simulink model "Experiment_cs"  (R2019a)
settings: Solver=ode5  StartTime=0.0  StopTime=inf  FixedStep=1/20  RelTol=1e-3
PreLoadFcn:
  | mbxruntime.callbacks.PreLoadFcn(bdroot);
PostLoadFcn:
  | mbxruntime.callbacks.PostLoadFcn(bdroot);
InitFcn:
  | mbxruntime.callbacks.InitFcn(bdroot);
StartFcn:
  | mbxruntime.callbacks.StartFcn(bdroot);
StopFcn:
  | mbxruntime.callbacks.StopFcn(bdroot);
model workspace: external: MAT-File .\Experiment_cs_hws.mat (data not in the file)
undefined symbols (not defined in the file or in its folder): DiscIntNeverNeededParam, Experiment_cs_BMW_X5_SUV_1_Dynamics_Empty_STATE_BMW_X5_SUV_1_x0, Experiment_cs_BMW_X5_SUV_1_Dynamics_Empty_STATE_BMW_X5_SUV_1_y0, Experiment_cs_BMW_X5_SUV_1_Dynamics_Empty_STATE_BMW_X5_SUV_1_z0, Experiment_cs_e1d584482631291c, Experiment_cs_e726c63043403dc7, Experiment_cs_f4cae83923a86e0b, InitImageOutputDir
libraries: adeye_lib x26, PreScanSimulinkLibrary x2, robotlib x1, PreScanUsefulBlocks x1
(part 1 of 2)
CloseFcn:
  | mbxruntime.callbacks.CloseFcn(bdroot);
settings Model: Creator=PRESCAN  LastModifiedBy=adeye
settings DataIOCC: LimitDataPoints=on  SaveFormat=Array  SignalLoggingSaveFormat=ModelDataLogs  ReturnWorkspaceOutputs=off
settings OptimizationCC: DefaultParameterBehavior=Inlined  ExpressionDepthLimit=2147483647  InitFltsAndDblsToZero=on  LifeSpan=inf
settings DebuggingCC: SaveWithParameterizedLinksMsg=none  UnderspecifiedInitializationDetection=Classic  MergeDetectMultiDrivingBlocksExec=none  SignalResolutionControl=TryResolveAllWithWarning  MultiTaskDSMMsg=warning  MultiTaskCondExecSysMsg=none  FcnCallInpInsideContextMsg=warning  StateNameClashWarn=warning  SFUnexpectedBacktrackingDiag=warning  SFNoUnconditionalDefaultTransitionDiag=warning  SFExecutionAtInitializationDiag=none  ArithmeticOperatorsInVariantConditions=warning
settings HardwareCC: ProdBitPerPointer=32  ProdBitPerSizeT=32  ProdBitPerPtrDiffT=32  ProdLargestAtomicFloat=None  ProdIntDivRoundTo=Undefined  ProdEndianess=Unspecified  ProdWordSize=32  ProdHWDeviceType=32-bit Generic
settings ModelReferenceCC: UpdateModelReferenceTargets=IfOutOfDate  PropagateSignalLabelsOutOfModel=off
settings SFSimCC: SimUseLocalCustomCode=off  SimParseCustomCode=off
settings SFSimCC: SimCustomHeaderCode=|
  | #include "prescan.h"
  | #include "prescan_platform.h"
settings RTWCC: RTWUseLocalCustomCode=off
settings CodeAppCC: StateflowObjectComments=on
settings GRTTargetCC: TargetFcnLib=ansi_tfl_tmw.mat  TargetLangStandard=C89/C90 (ANSI)  GeneratePreprocessorConditionals=Disable all  CombineOutputUpdateFcns=off  GRTInterface=on
settings ConfigComp: CovMetricSettings=dw  CovHtmlReporting=on  CovSaveCumulativeToWorkspaceVar=on  CovSaveSingleToWorkspaceVar=on  CovExternalEMLEnable=off  CovSFcnEnable=off

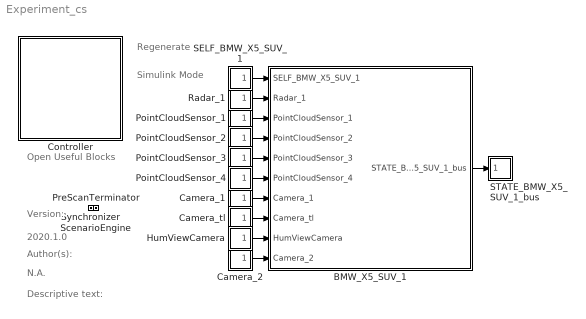
== system Experiment_cs ==
  note: Regenerate
  note: Simulink Mode
  note: Open Useful Blocks
  note: 2020.1.0
  note: Version:
  note: Author(s):
  note: N.A.
  note: Descriptive text:
  BMW_X5_SUV_1 : Subsystem  Tag=WorldObjectSubSystem  InitFcn=UniqueId = '256';
      mask init:
      | modelPath = GenericModelHelper.getGenericModelFilePath('ModelDepo','Vehicles\BMW_X5\BMW_X5.pgmb','bfeb1c11467705ab888b3011684c848b');imagePath = GenericModelHelper.getCompilationPicture(modelPath, 'BMW_X5_HighPoly.png');
      mask Display: image(imread(imagePath));color('white');text(0, 0, ' ID=14\n')
  Camera_1 : Subsystem  Tag=sensor/Camera/CameraSensor  Priority=30  mask(PreScan Source Block: Camera Sensor){}
      mask help: The Camera Sensor provides a color or monochrome image.
      settings: OpenFcn=open_system([gcb '/Sensor'],'mask')
      mask Help: eval('openHelp(457)')
      mask Display: image(imread('CameraSensor.png'))
  Camera_2 : Subsystem  Tag=sensor/Camera/CameraSensor  Priority=30  mask(PreScan Source Block: Camera Sensor){}
      mask help: The Camera Sensor provides a color or monochrome image.
      settings: OpenFcn=open_system([gcb '/Sensor'],'mask')
      mask Help: eval('openHelp(457)')
      mask Display: image(imread('CameraSensor.png'))
  Camera_tl : Subsystem  Tag=sensor/Camera/CameraSensor  Priority=30  mask(PreScan Source Block: Camera Sensor){}
      mask help: The Camera Sensor provides a color or monochrome image.
      settings: OpenFcn=open_system([gcb '/Sensor'],'mask')
      mask Help: eval('openHelp(457)')
      mask Display: image(imread('CameraSensor.png'))
  Controller : Subsystem  Description=8A3CD2955739A82C886C20AE3E253D78460D53180EE2C1B14CC08DF75A70BE77  Priority=-1  LoadFcn=load PreScanControllerData  mask(PreScan Simulation Controller){prescanversion='2020.1.0', ModelReferencing=off, TimeStep=1/20, ControlMode=0, PreScanExecutionMode=on, ControllerCount=0, ControllerIndex=0, ControllerOptions=''}
      mask prompts: prescanversion "PreScan Version"; ModelReferencing "Use Model Referencing"; TimeStep "Upload Period [s]"; ControlMode "Control Mode"; PreScanExecutionMode "Execution Mode"; ControllerCount "Controller Count"; ControllerIndex "Controller Index"; ControllerOptions "Controller Options"
      mask help:
      | Please do not remove this block from the compilation sheet,
      | as it connects the model to the PreScan environment.
      mask init:
      | model = bdroot(gcb);
      | ExperimentFile = mbxruntime.findExperimentFile(model,true); %relative path
      | 
      | [d1, d2, d3, prescandata] = prescan_Settings();
      | ModelDepo = fullfile(prescandata,'ModelDepo'); 
      | 
      | RTmode = mbxruntime.getRTMode(model);
      | 
      | SimulationMode = get_param(bdroot,'SimulationMode');
      | if strcmp(SimulationMode, 'rapid-accelerator')
      |     SimulationMode = 'external';
      | end
      | TargetName = get_param(bdroot,'SystemTargetFile');
      settings: ModelCloseFcn=assignin('base',['model_closed_' bdroot],true);
      mask Help: eval('openHelp(812)')
      mask Display: image(imread('prescanlogo.ico'))
  HumViewCamera : Subsystem  Tag=sensor/Camera/CameraSensor  Priority=30  mask(PreScan Source Block: Camera Sensor){}
      mask help: The Camera Sensor provides a color or monochrome image.
      settings: OpenFcn=open_system([gcb '/Sensor'],'mask')
      mask Help: eval('openHelp(457)')
      mask Display: image(imread('CameraSensor.png'))
  PointCloudSensor_1 : Subsystem  Tag=sensor/PointCloudInport  Priority=30  mask(PreScan Source Block: Point Cloud Sensor){}
      mask help: The Point Cloud Sensor provides XYZ positions relative to the sensor
      settings: OpenFcn=open_system([gcb '/Sensor'],'mask')
      mask Help: eval('openHelp(6400)')
      mask Display: image(imread('PointCloudSensorSL.png'))
  PointCloudSensor_2 : Subsystem  Tag=sensor/PointCloudInport  Priority=30  mask(PreScan Source Block: Point Cloud Sensor){}
      mask help: The Point Cloud Sensor provides XYZ positions relative to the sensor
      settings: OpenFcn=open_system([gcb '/Sensor'],'mask')
      mask Help: eval('openHelp(6400)')
      mask Display: image(imread('PointCloudSensorSL.png'))
  PointCloudSensor_3 : Subsystem  Tag=sensor/PointCloudInport  Priority=30  mask(PreScan Source Block: Point Cloud Sensor){}
      mask help: The Point Cloud Sensor provides XYZ positions relative to the sensor
      settings: OpenFcn=open_system([gcb '/Sensor'],'mask')
      mask Help: eval('openHelp(6400)')
      mask Display: image(imread('PointCloudSensorSL.png'))
  PointCloudSensor_4 : Subsystem  Tag=sensor/PointCloudInport  Priority=30  mask(PreScan Source Block: Point Cloud Sensor){}
      mask help: The Point Cloud Sensor provides XYZ positions relative to the sensor
      settings: OpenFcn=open_system([gcb '/Sensor'],'mask')
      mask Help: eval('openHelp(6400)')
      mask Display: image(imread('PointCloudSensorSL.png'))
  PreScanTerminator : Subsystem  Tag=PreScanTerminator  Priority=999  LoadFcn=load PrescanTerminatorData  mask(PreScan Simulation Terminator){TimeStep=1/20}
      mask prompts: TimeStep "Upload Period [s]"
      mask help:
      | Please do not remove this block from the compilation sheet as it
      | connects the model to the PreScan environment.
      mask Help: eval('openHelp(812)')
      mask Display: image(imread('prescanlogo.ico'))
  Radar_1 : Subsystem  Tag=sensor/Radar  Priority=30  LoadFcn=load('PrescanScannerSensorData.mat');load('PrescanScannerSensorMessage.mat')  mask(PreScan Source Block: Radar Sensor){}
      mask help:
      | The Radar Sensor is a detailed sensor based on a physical radar
      | model that includes Antenna GAIN Maps (AGM) and atmospheric
      | attenuation.
      |
      | For more information, please click Help.
      settings: OpenFcn=open_system([gcb '/Sensor'],'mask')
      mask Help: eval('openHelp(1464)')
      mask Display: image(imread('Radar.png'))
  SELF_BMW_X5_SUV_1 : Subsystem  Tag=sensor/SelfPort  Priority=30  LoadFcn=load('PreScanSelfSensorData.mat')  mask(PreScan Source Block: SELF){}
      mask help:
      | The SELF port shows (state) information of the actor itself. The outputs are position in the experiment's axis system and the GPS coordinates, and the object's absolute velocity and compass heading.
      |
      | For more information, please click Help.
      settings: OpenFcn=open_system([gcb '/Sensor'],'mask')
      mask Help: eval('openHelp(462)')
      mask Display: image(imread('GPS.png'))
  STATE_BMW_X5_SUV_1_bus : Subsystem  Tag=actuator/StatePort  Priority=0  LoadFcn=load('PreScanStateActuatorData.mat')  mask(PreScan Sink Block: State){}
      mask help:
      | The Actor State contains a vector signal of size (9x1), containing the following signals:
      |
      | -  Position    	(x,y,z)             	[m]
      | -  Velocity    	(vx,vy,vz)         	[m/s]
      | -  Angles       	(Roll, Pitch, Yaw)	[rad]
      |
      | The Actor state is defined in the global axis system.
      | The state is superponed on the Initial position defined in the GUI.
      |
      | For more information, please click Help.
      settings: OpenFcn=open_system([gcb '/Actuator'],'mask')
      mask Help: eval('openHelp(222)')
      mask Display: image(imread('State.png'))
  ScenarioEngine : Subsystem  Tag=PreScanOpenScenarioBlock  Priority=10  LoadFcn=load PrescanSynchronizeData  mask(PreScan Simulation Core Block){TimeStep=1/20}
      mask prompts: TimeStep "Timestep [s]"
      mask help:
      | Please do not remove this block from the PreScan compilation sheet,
      | as it contains essential configuration parameters for a PreScan simulation.
      settings: DeleteFcn=PreScanBlockDeleteFcn;
      mask Display: image(imread('prescanlogo.ico'))
  Synchronizer : Subsystem  Tag=PreScanSynchronizer  Priority=20  LoadFcn=load PrescanSynchronizeData  mask(PreScan Simulation Core Block){TimeStep=1/20}
      mask prompts: TimeStep "Timestep [s]"
      mask help:
      | Please do not remove this block from the PreScan compilation sheet,
      | as it contains essential configuration parameters for a PreScan simulation.
      settings: DeleteFcn=PreScanBlockDeleteFcn;
      mask Display: image(imread('prescanlogo.ico'))
  wires:
  BMW_X5_SUV_1/1(STATE_BMW_X5_SUV_1_bus) -> STATE_BMW_X5_SUV_1_bus/1(STATE_BMW_X5_SUV_1_bus)
  SELF_BMW_X5_SUV_1/1(SELF_BMW_X5_SUV_1) -> BMW_X5_SUV_1/1(SELF_BMW_X5_SUV_1)
  Radar_1/1(Radar_1) -> BMW_X5_SUV_1/2(Radar_1)
  PointCloudSensor_1/1(PointCloudSensor_1) -> BMW_X5_SUV_1/3(PointCloudSensor_1)
  PointCloudSensor_2/1(PointCloudSensor_2) -> BMW_X5_SUV_1/4(PointCloudSensor_2)
  PointCloudSensor_3/1(PointCloudSensor_3) -> BMW_X5_SUV_1/5(PointCloudSensor_3)
  PointCloudSensor_4/1(PointCloudSensor_4) -> BMW_X5_SUV_1/6(PointCloudSensor_4)
  Camera_1/1(Camera_1) -> BMW_X5_SUV_1/7(Camera_1)
  Camera_tl/1(Camera_tl) -> BMW_X5_SUV_1/8(Camera_tl)
  HumViewCamera/1(HumViewCamera) -> BMW_X5_SUV_1/9(HumViewCamera)
  Camera_2/1(Camera_2) -> BMW_X5_SUV_1/10(Camera_2)

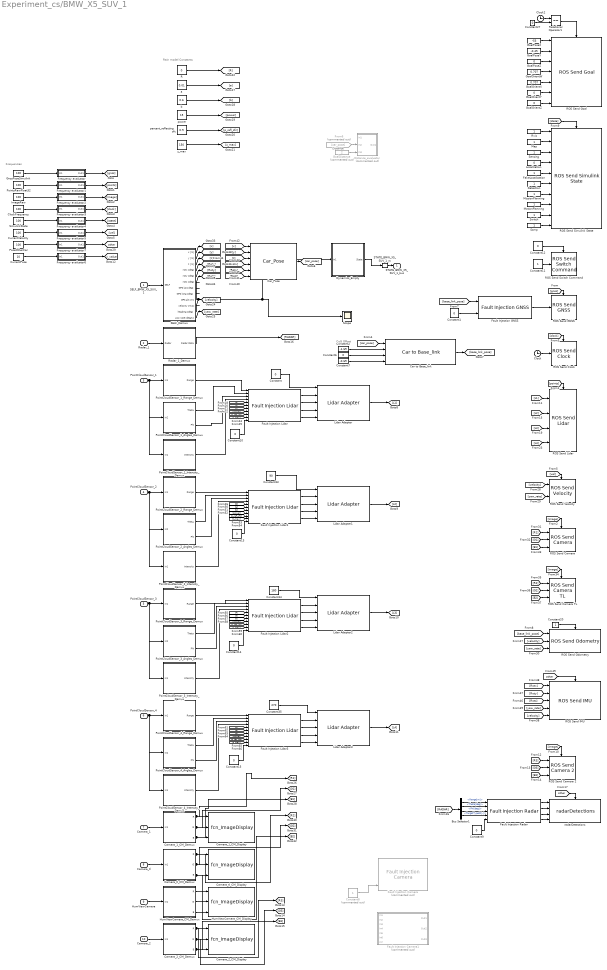
== system Experiment_cs/BMW_X5_SUV_1 ==
  note: Distance
  note: Frequencies
  note: CoG Offset
  note: Rain model Constants
  SELF_BMW_X5_SUV_1 : Inport  Tag=inport/SelfPort  OutDataTypeStr=Bus: PRESCAN_SELFSENSORDATA  PortDimensions=1  SampleTime=1/20  BusOutputAsStruct=on
  Radar_1 : Inport  Tag=inport/Radar  Port=2  OutDataTypeStr=Bus: PRESCAN_SCANNERSENSOR_MESSAGE  PortDimensions=7  SampleTime=1/20  BusOutputAsStruct=on
  PointCloudSensor_1 : Inport  Tag=inport/PointCloudInport  Port=3  OutDataTypeStr=single  SampleTime=1/20  BusOutputAsStruct=on
  PointCloudSensor_2 : Inport  Tag=inport/PointCloudInport  Port=4  OutDataTypeStr=single  SampleTime=1/20  BusOutputAsStruct=on
  PointCloudSensor_3 : Inport  Tag=inport/PointCloudInport  Port=5  OutDataTypeStr=single  SampleTime=1/20  BusOutputAsStruct=on
  PointCloudSensor_4 : Inport  Tag=inport/PointCloudInport  Port=6  OutDataTypeStr=single  SampleTime=1/20  BusOutputAsStruct=on
  Camera_1 : Inport  Tag=inport/Camera/CameraSensor  Port=7  OutDataTypeStr=uint8  SampleTime=1/20  BusOutputAsStruct=on
  Camera_tl : Inport  Tag=inport/Camera/CameraSensor  Port=8  OutDataTypeStr=uint8  SampleTime=1/20  BusOutputAsStruct=on
  HumViewCamera : Inport  Tag=inport/Camera/CameraSensor  Port=9  OutDataTypeStr=uint8  SampleTime=1/20  BusOutputAsStruct=on
  Camera_2 : Inport  Tag=inport/Camera/CameraSensor  Port=10  OutDataTypeStr=uint8  SampleTime=1/20  BusOutputAsStruct=on
  Bus Selector1 : BusSelector  OutputSignals=Range[m],Theta[deg],Phi[deg],TargetTypeID[-]
  Camera_1_CM_Demux : Subsystem  Tag=demux/Camera/Color  mask{SensorName=Camera_1, hres=960, vres=720}
      mask prompts: SensorName "Sensor Name"; hres "Horizontal Resolution"; vres "Vertical Resolution"
      mask Help: eval('openHelp(457)')
      mask Display:
      | fprintf('MONO CAMERA:\n Color\n %s \n %d x %d px',SensorName,hres,vres)
      | port_label('output',1,'R')
      | port_label('output',2,'G')
      | port_label('output',3,'B')
  Camera_1_CM_Display : M-S-Function  Tag=CameraSensor_Color_Display  InitFcn=InitImageOutputDir(gcb);  FunctionName=fcn_ImageDisplay  Parameters=SensorName EnableDisplay EnablePosition DisplayPosition FigureHandle SaveResults BitmapFormat TempOutputDir CameraType DataType  mask(PreScan Color Display Block){SensorName=Camera_1, EnableDisplay=on, EnablePosition=off, DisplayPosition=[10 10 960 720], FigureHandle=25605, SaveResults=off, Format=PNG, TempOutputDir=0, CameraType=Mono, DataType=uint8}
      mask prompts: SensorName "User Specified: Title of Display"; EnableDisplay "Active"; EnablePosition "Set Display window position"; DisplayPosition "Display window position [xpos ypos width height]"; FigureHandle "Unique Handle"; SaveResults "Save results"; TempOutputDir "OutputDir"; CameraType "Camera Type"; DataType "Image Data Type"
      mask help: This block displays the RGB output of a PreScan camera sensor.
      mask init:
      | if EnableDisplay
      |     EnableString='';
      |     EnableColor='gray';
      | else
      |     EnableString='INACTIVE';
      |     EnableColor='red';
      | end
      | switch Format
      |     case 1
      |         BitmapFormat = 'png';
      |     case 2
      |         BitmapFormat = 'bmp';
      |     case 3
      |         BitmapFormat = 'jpg';
      | end 
      | if CameraType==1
      |     CameraTypeName='MONO';
      |     PortNumber=0;
      | else
      |     CameraTypeName='STEREO';
      |     PortNumber=3;
      | end
      settings: CopyFcn=CopyFcnDisplay  DeleteFcn=PreScanBlockDeleteFcn;  ModelCloseFcn=fcn_ImageDisplay_ModelCloseFcn
      mask Help: eval('openHelp(457)')
      mask Callback EnablePosition:
      | MV=get_param(gcb,'MaskVisibilities');
      | if strcmp(get_param(gcb,'EnablePosition'),'on')
      |     MV{4}='on';
      | else
      |     MV{4}='off';
      | end
      | set_param(gcb,'MaskVisibilities',MV);
      | clear MV;
      mask TypeOptions Format: PNG | BMP | JPG
      mask TypeOptions CameraType: Mono | Stereo
      mask TypeOptions DataType: uint8 | single
      mask Display:
      | color(EnableColor);
      | fprintf('%s\n DISPLAY:\n Color \n %s',EnableString,SensorName)
      | port_label('input',1,'R')
      | port_label('input',2,'G')
      | port_label('input',3,'B')
      | port_label('input',PortNumber+1,'R')
      | port_label('input',PortNumber+2,'G')
      | port_label('input',PortNumber+3,'B')
  Camera_2_CM_Demux : Subsystem  Tag=demux/Camera/Color  mask{SensorName=Camera_2, hres=960, vres=720}
      mask prompts: SensorName "Sensor Name"; hres "Horizontal Resolution"; vres "Vertical Resolution"
      mask Help: eval('openHelp(457)')
      mask Display:
      | fprintf('MONO CAMERA:\n Color\n %s \n %d x %d px',SensorName,hres,vres)
      | port_label('output',1,'R')
      | port_label('output',2,'G')
      | port_label('output',3,'B')
  Camera_2_CM_Display : M-S-Function  Tag=CameraSensor_Color_Display  InitFcn=InitImageOutputDir(gcb);  FunctionName=fcn_ImageDisplay  Parameters=SensorName EnableDisplay EnablePosition DisplayPosition FigureHandle SaveResults BitmapFormat TempOutputDir CameraType DataType  mask(PreScan Color Display Block){SensorName=Camera_2, EnableDisplay=on, EnablePosition=off, DisplayPosition=[10 10 960 720], FigureHandle=25608, SaveResults=off, Format=PNG, TempOutputDir=0, CameraType=Mono, DataType=uint8}
      mask prompts: SensorName "User Specified: Title of Display"; EnableDisplay "Active"; EnablePosition "Set Display window position"; DisplayPosition "Display window position [xpos ypos width height]"; FigureHandle "Unique Handle"; SaveResults "Save results"; TempOutputDir "OutputDir"; CameraType "Camera Type"; DataType "Image Data Type"
      mask help: This block displays the RGB output of a PreScan camera sensor.
      mask init: same as Experiment_cs/BMW_X5_SUV_1/Camera_1_CM_Display
      settings: CopyFcn=CopyFcnDisplay  DeleteFcn=PreScanBlockDeleteFcn;  ModelCloseFcn=fcn_ImageDisplay_ModelCloseFcn
      mask Help: eval('openHelp(457)')
      mask Callback EnablePosition:
      | MV=get_param(gcb,'MaskVisibilities');
      | if strcmp(get_param(gcb,'EnablePosition'),'on')
      |     MV{4}='on';
      | else
      |     MV{4}='off';
      | end
      | set_param(gcb,'MaskVisibilities',MV);
      | clear MV;
      mask TypeOptions Format: PNG | BMP | JPG
      mask TypeOptions CameraType: Mono | Stereo
      mask TypeOptions DataType: uint8 | single
      mask Display:
      | color(EnableColor);
      | fprintf('%s\n DISPLAY:\n Color \n %s',EnableString,SensorName)
      | port_label('input',1,'R')
      | port_label('input',2,'G')
      | port_label('input',3,'B')
      | port_label('input',PortNumber+1,'R')
      | port_label('input',PortNumber+2,'G')
      | port_label('input',PortNumber+3,'B')
  Camera_tl_CM_Demux : Subsystem  Tag=demux/Camera/Color  mask{SensorName=Camera_tl, hres=960, vres=720}
      mask prompts: SensorName "Sensor Name"; hres "Horizontal Resolution"; vres "Vertical Resolution"
      mask Help: eval('openHelp(457)')
      mask Display:
      | fprintf('MONO CAMERA:\n Color\n %s \n %d x %d px',SensorName,hres,vres)
      | port_label('output',1,'R')
      | port_label('output',2,'G')
      | port_label('output',3,'B')
  Camera_tl_CM_Display : M-S-Function  Tag=CameraSensor_Color_Display  InitFcn=InitImageOutputDir(gcb);  FunctionName=fcn_ImageDisplay  Parameters=SensorName EnableDisplay EnablePosition DisplayPosition FigureHandle SaveResults BitmapFormat TempOutputDir CameraType DataType  mask(PreScan Color Display Block){SensorName=Camera_tl, EnableDisplay=on, EnablePosition=off, DisplayPosition=[10 10 960 720], FigureHandle=25606, SaveResults=off, Format=PNG, TempOutputDir=0, CameraType=Mono, DataType=uint8}
      mask prompts: SensorName "User Specified: Title of Display"; EnableDisplay "Active"; EnablePosition "Set Display window position"; DisplayPosition "Display window position [xpos ypos width height]"; FigureHandle "Unique Handle"; SaveResults "Save results"; TempOutputDir "OutputDir"; CameraType "Camera Type"; DataType "Image Data Type"
      mask help: This block displays the RGB output of a PreScan camera sensor.
      mask init: same as Experiment_cs/BMW_X5_SUV_1/Camera_1_CM_Display
      settings: CopyFcn=CopyFcnDisplay  DeleteFcn=PreScanBlockDeleteFcn;  ModelCloseFcn=fcn_ImageDisplay_ModelCloseFcn
      mask Help: eval('openHelp(457)')
      mask Callback EnablePosition:
      | MV=get_param(gcb,'MaskVisibilities');
      | if strcmp(get_param(gcb,'EnablePosition'),'on')
      |     MV{4}='on';
      | else
      |     MV{4}='off';
      | end
      | set_param(gcb,'MaskVisibilities',MV);
      | clear MV;
      mask TypeOptions Format: PNG | BMP | JPG
      mask TypeOptions CameraType: Mono | Stereo
      mask TypeOptions DataType: uint8 | single
      mask Display:
      | color(EnableColor);
      | fprintf('%s\n DISPLAY:\n Color \n %s',EnableString,SensorName)
      | port_label('input',1,'R')
      | port_label('input',2,'G')
      | port_label('input',3,'B')
      | port_label('input',PortNumber+1,'R')
      | port_label('input',PortNumber+2,'G')
      | port_label('input',PortNumber+3,'B')
  Car to Base_link : adeye_lib/Car to Base_link  SystemSampleTime=-1
  Car_Pose : adeye_lib/Car_Pose  SystemSampleTime=-1
  Clock : Clock
  Clock2 : Clock
  ClockFrequency : Constant  Value=100
  Constant{,10,13..15} (5 alike) : Constant  Value=0  OutDataTypeStr=Inherit: Inherit via back propagation
  Constant1 : Constant  Value=0  OutDataTypeStr=Inherit: Inherit via back propagation  SampleTime=0.05
  Constant11 : Constant  OutDataTypeStr=Inherit: Inherit via back propagation  SampleTime=0.05
  Constant12 : Constant  Value=0  OutDataTypeStr=Inherit: Inherit via back propagation  SampleTime=0.05
  Constant2 : Constant  Value=-1.69
  Constant20 : Constant
  Constant27 : Constant  Value=0
  Constant33 : Constant  Value=90  OutDataTypeStr=Inherit: Inherit via back propagation
  Constant34 : Constant  Value=180  OutDataTypeStr=Inherit: Inherit via back propagation
  Constant35 : Constant  Value=270  OutDataTypeStr=Inherit: Inherit via back propagation
  Constant6 : Constant  Value=0
  Constant7 : Constant  Value=-0.69
  Constant8 : Constant  Commented=on
  Constant9 : Constant  Value=0
  CurrentPose : Constant  Value=10
  CurrentVelocity : Constant  Value=100
  Detection : Constant
  Distance_evaluator : Subsystem  Commented=on
  Dynamics_Empty : Subsystem  Tag=Dynamics_Empty
      mask Help: eval('openHelp(202)')
      mask Display: port_label('output', 1, 'State');text(0,0,' Empty\n')
  FakeLocalization : Constant
  Fault Injection Camera : adeye_lib/Fault Injection Camera  Commented=on  idy=200  idx=100  x=100  y=150  R=0  G=0  B=0
  Fault Injection Camera1 : Subsystem  Commented=on
      mask Display:
      | fprintf('Fault inj\n Camera\n')
      | 
      | port_label('input',1,'dx')
      | port_label('input',2,'dy')
      | port_label('input',3,'Error')
      | port_label('input',4,'R')
      | port_label('input',5,'G')
      | port_label('input',6,'B')
      | port_label('input',7,'On/Off')
      | 
      | port_label('output',1,'R')
      | port_label('output',2,'G')
      | port_label('output',3,'B')
  Fault Injection GNSS : adeye_lib/Fault Injection GNSS  v=0.0001  f=20
  Fault Injection Lidar{,1..3} (4 alike) : adeye_lib/Fault Injection Lidar  vr=0.0001  vi=0.0001  f=20  p=225*16
  Fault Injection Radar : adeye_lib/Fault Injection Radar  n=7  vr=1  vt=1  vp=1
  Frequency evaluator : Subsystem
  Frequency evaluator1 : Subsystem
  Frequency evaluator2 : Subsystem
  Frequency evaluator3 : Subsystem
  Frequency evaluator4 : Subsystem
  Frequency evaluator5 : Subsystem
  Frequency evaluator6 : Subsystem
  Frequency evaluator7 : Subsystem
  From6 : From  Commented=on  GotoTag=car_pose
  GnssPoseSimulink : Constant  Value=100
  GoalDistance : Constant  Commented=on  Value=2
  GoalOrientW : Constant  Value=0.707
  GoalOrientX : Constant  Value=0.707
  GoalOrientY : Constant  Value=0
  GoalOrientZ : Constant  Value=0
  GoalPoseX : Constant  Value=-53
  GoalPoseY : Constant  Value=-0.45
  GoalPoseZ : Constant  Value=0
  HumViewCamera_CM_Demux : Subsystem  Tag=demux/Camera/Color  mask{SensorName=HumViewCamera, hres=1871, vres=1080}
      mask prompts: SensorName "Sensor Name"; hres "Horizontal Resolution"; vres "Vertical Resolution"
      mask Help: eval('openHelp(457)')
      mask Display:
      | fprintf('MONO CAMERA:\n Color\n %s \n %d x %d px',SensorName,hres,vres)
      | port_label('output',1,'R')
      | port_label('output',2,'G')
      | port_label('output',3,'B')
  HumViewCamera_CM_Display : M-S-Function  Tag=CameraSensor_Color_Display  InitFcn=InitImageOutputDir(gcb);  FunctionName=fcn_ImageDisplay  Parameters=SensorName EnableDisplay EnablePosition DisplayPosition FigureHandle SaveResults BitmapFormat TempOutputDir CameraType DataType  mask(PreScan Color Display Block){SensorName=HumViewCamera, EnableDisplay=on, EnablePosition=off, DisplayPosition=[10 10 1871 1080], FigureHandle=25607, SaveResults=off, Format=PNG, TempOutputDir=0, CameraType=Mono, DataType=uint8}
      mask prompts: SensorName "User Specified: Title of Display"; EnableDisplay "Active"; EnablePosition "Set Display window position"; DisplayPosition "Display window position [xpos ypos width height]"; FigureHandle "Unique Handle"; SaveResults "Save results"; TempOutputDir "OutputDir"; CameraType "Camera Type"; DataType "Image Data Type"
      mask help: This block displays the RGB output of a PreScan camera sensor.
      mask init: same as Experiment_cs/BMW_X5_SUV_1/Camera_1_CM_Display
      settings: CopyFcn=CopyFcnDisplay  DeleteFcn=PreScanBlockDeleteFcn;  ModelCloseFcn=fcn_ImageDisplay_ModelCloseFcn
      mask Help: eval('openHelp(457)')
      mask Callback EnablePosition:
      | MV=get_param(gcb,'MaskVisibilities');
      | if strcmp(get_param(gcb,'EnablePosition'),'on')
      |     MV{4}='on';
      | else
      |     MV{4}='off';
      | end
      | set_param(gcb,'MaskVisibilities',MV);
      | clear MV;
      mask TypeOptions Format: PNG | BMP | JPG
      mask TypeOptions CameraType: Mono | Stereo
      mask TypeOptions DataType: uint8 | single
      mask Display:
      | color(EnableColor);
      | fprintf('%s\n DISPLAY:\n Color \n %s',EnableString,SensorName)
      | port_label('input',1,'R')
      | port_label('input',2,'G')
      | port_label('input',3,'B')
      | port_label('input',PortNumber+1,'R')
      | port_label('input',PortNumber+2,'G')
      | port_label('input',PortNumber+3,'B')
  ImageRaw : Constant  Value=100
  Lidar Adapter{,1..3} (4 alike) : adeye_lib/Lidar Adapter  SystemSampleTime=-1
  Localization : Constant  Value=0
  Map : Constant
  MissionPlanning : Constant
  MotionPlanning : Constant
  PointCloudSensor_1_Angles_Demux : Subsystem  Tag=demux/PCS/Angles  mask{SensorName=PointCloudSensor_1, offset=225, hres=225, vres=16}
      mask prompts: SensorName "Sensor Name"; offset "Data Start"; hres "Horizontal Resolution"; vres "Vertical Resolution"
      mask Help: eval('openHelp(6400)')
      mask Display:
      | fprintf('Point Cloud:\n Data\n %s \n %d x %d px',SensorName,hres,vres)
      | port_label('output',1,'Theta')
      | port_label('output',2,'Phi')
  PointCloudSensor_1_Intensity_Demux : Subsystem  Tag=demux/PCS/Intensity  mask{SensorName=PointCloudSensor_1, offset=675, hres=225, vres=16}
      mask prompts: SensorName "Sensor Name"; offset "Data Start"; hres "Horizontal Resolution"; vres "Vertical Resolution"
      mask Help: eval('openHelp(6400)')
      mask Display:
      | fprintf('Point Cloud:\n Data\n %s \n %d x %d px',SensorName,hres,vres)
      | port_label('output',1,'Intensity')
  PointCloudSensor_1_Range_Demux : Subsystem  Tag=demux/PCS/Range  mask{SensorName=PointCloudSensor_1, offset=0, hres=225, vres=16}
      mask prompts: SensorName "Sensor Name"; offset "Data Start"; hres "Horizontal Resolution"; vres "Vertical Resolution"
      mask Help: eval('openHelp(6400)')
      mask Display:
      | fprintf('Point Cloud:\n Data\n %s \n %d x %d px',SensorName,hres,vres)
      | port_label('output',1,'Range')
  PointCloudSensor_2_Angles_Demux : Subsystem  Tag=demux/PCS/Angles  mask{SensorName=PointCloudSensor_2, offset=225, hres=225, vres=16}
      mask prompts: SensorName "Sensor Name"; offset "Data Start"; hres "Horizontal Resolution"; vres "Vertical Resolution"
      mask Help: eval('openHelp(6400)')
      mask Display:
      | fprintf('Point Cloud:\n Data\n %s \n %d x %d px',SensorName,hres,vres)
      | port_label('output',1,'Theta')
      | port_label('output',2,'Phi')
  PointCloudSensor_2_Intensity_Demux : Subsystem  Tag=demux/PCS/Intensity  mask{SensorName=PointCloudSensor_2, offset=675, hres=225, vres=16}
      mask prompts: SensorName "Sensor Name"; offset "Data Start"; hres "Horizontal Resolution"; vres "Vertical Resolution"
      mask Help: eval('openHelp(6400)')
      mask Display:
      | fprintf('Point Cloud:\n Data\n %s \n %d x %d px',SensorName,hres,vres)
      | port_label('output',1,'Intensity')
  PointCloudSensor_2_Range_Demux : Subsystem  Tag=demux/PCS/Range  mask{SensorName=PointCloudSensor_2, offset=0, hres=225, vres=16}
      mask prompts: SensorName "Sensor Name"; offset "Data Start"; hres "Horizontal Resolution"; vres "Vertical Resolution"
      mask Help: eval('openHelp(6400)')
      mask Display:
      | fprintf('Point Cloud:\n Data\n %s \n %d x %d px',SensorName,hres,vres)
      | port_label('output',1,'Range')
  PointCloudSensor_3_Angles_Demux : Subsystem  Tag=demux/PCS/Angles  mask{SensorName=PointCloudSensor_3, offset=225, hres=225, vres=16}
      mask prompts: SensorName "Sensor Name"; offset "Data Start"; hres "Horizontal Resolution"; vres "Vertical Resolution"
      mask Help: eval('openHelp(6400)')
      mask Display:
      | fprintf('Point Cloud:\n Data\n %s \n %d x %d px',SensorName,hres,vres)
      | port_label('output',1,'Theta')
      | port_label('output',2,'Phi')
  PointCloudSensor_3_Intensity_Demux : Subsystem  Tag=demux/PCS/Intensity  mask{SensorName=PointCloudSensor_3, offset=675, hres=225, vres=16}
      mask prompts: SensorName "Sensor Name"; offset "Data Start"; hres "Horizontal Resolution"; vres "Vertical Resolution"
      mask Help: eval('openHelp(6400)')
      mask Display:
      | fprintf('Point Cloud:\n Data\n %s \n %d x %d px',SensorName,hres,vres)
      | port_label('output',1,'Intensity')
  PointCloudSensor_3_Range_Demux : Subsystem  Tag=demux/PCS/Range  mask{SensorName=PointCloudSensor_3, offset=0, hres=225, vres=16}
      mask prompts: SensorName "Sensor Name"; offset "Data Start"; hres "Horizontal Resolution"; vres "Vertical Resolution"
      mask Help: eval('openHelp(6400)')
      mask Display:
      | fprintf('Point Cloud:\n Data\n %s \n %d x %d px',SensorName,hres,vres)
      | port_label('output',1,'Range')
  PointCloudSensor_4_Angles_Demux : Subsystem  Tag=demux/PCS/Angles  mask{SensorName=PointCloudSensor_4, offset=225, hres=225, vres=16}
      mask prompts: SensorName "Sensor Name"; offset "Data Start"; hres "Horizontal Resolution"; vres "Vertical Resolution"
      mask Help: eval('openHelp(6400)')
      mask Display:
      | fprintf('Point Cloud:\n Data\n %s \n %d x %d px',SensorName,hres,vres)
      | port_label('output',1,'Theta')
      | port_label('output',2,'Phi')
  PointCloudSensor_4_Intensity_Demux : Subsystem  Tag=demux/PCS/Intensity  mask{SensorName=PointCloudSensor_4, offset=675, hres=225, vres=16}
      mask prompts: SensorName "Sensor Name"; offset "Data Start"; hres "Horizontal Resolution"; vres "Vertical Resolution"
      mask Help: eval('openHelp(6400)')
      mask Display:
      | fprintf('Point Cloud:\n Data\n %s \n %d x %d px',SensorName,hres,vres)
      | port_label('output',1,'Intensity')
  PointCloudSensor_4_Range_Demux : Subsystem  Tag=demux/PCS/Range  mask{SensorName=PointCloudSensor_4, offset=0, hres=225, vres=16}
      mask prompts: SensorName "Sensor Name"; offset "Data Start"; hres "Horizontal Resolution"; vres "Vertical Resolution"
      mask Help: eval('openHelp(6400)')
      mask Display:
      | fprintf('Point Cloud:\n Data\n %s \n %d x %d px',SensorName,hres,vres)
      | port_label('output',1,'Range')
  PointsRawFloat32 : Constant  Value=100
  PoseOtherCar : Constant  Value=100
  R : Constant  Value=0
  ROS Send Camera : adeye_lib/ROS Send Camera  SystemSampleTime=-1
  ROS Send Camera 2 : adeye_lib/ROS Send Camera 2  SystemSampleTime=-1
  ROS Send Camera TL : adeye_lib/ROS Send Camera TL  SystemSampleTime=-1
  ROS Send Clock : adeye_lib/ROS Send Clock  SystemSampleTime=-1
  ROS Send GNSS : adeye_lib/ROS Send GNSS  SystemSampleTime=-1
  ROS Send Goal : adeye_lib/ROS Send Goal  SystemSampleTime=-1
  ROS Send IMU : adeye_lib/ROS Send IMU  SystemSampleTime=-1
  ROS Send Lidar : adeye_lib/ROS Send Lidar  SystemSampleTime=-1
  ROS Send Odometry : adeye_lib/ROS Send Odometry  SystemSampleTime=-1
  ROS Send Simulink State : adeye_lib/ROS Send Simulink State  SystemSampleTime=-1
  ROS Send Switch Command : adeye_lib/ROS Send Switch Command  SystemSampleTime=-1
  ROS Send Velocity : adeye_lib/ROS Send Velocity  SystemSampleTime=-1
  Radar_1_Demux : Subsystem  Tag=demux/Radar  TreatAsAtomicUnit=on  mask(PreScan Demux Block: Radar){MAXMESSAGES=7}
      mask prompts: MAXMESSAGES "Number of Objects"
      mask help:
      | The Radar Sensor is a detailed sensor based on a physical radar
      | model that includes Antenna GAIN Maps (AGM) and atmospheric
      | attenuation.
      |
      | For more information, please click Help.
      mask Help: eval('openHelp(1464)')
      mask Display:
      | port_label('input',1,'Radar')
      | port_label('output',1,'Radar Data')
  Relational Operator1 : RelationalOperator  Operator===  OutDataTypeStr=boolean  RndMeth=Simplest
  Rviz : Constant
  SELF_Demux : Subsystem  Tag=demux/SelfPort  mask(PreScan Demux Block:){}
      mask help:
      | The SELF port shows (state) information of the actor itself. The outputs are position in the experiment's axis system and the GPS coordinates, and the object's absolute velocity and compass heading.
      |
      | For more information, please click Help.
      settings: DeleteFcn=PreScanBlockDeleteFcn;
      mask Help: eval('openHelp(462)')
      mask Display:
      | port_label('output',1,'x [m]')
      | port_label('output',2,'y [m]')
      | port_label('output',3,'z [m]','texmode','on')
      | port_label('output',4,'Rotx [deg]','texmode','on')
      | port_label('output',5,'Roty [deg]','texmode','on')
      | port_label('output',6,'Rotz [deg]','texmode','on')
      | port_label('output',7,'GPS lat [deg]','texmode','on')
      | port_label('output',8,'GPS long [deg]','texmode','on')
      | port_label('output',9,'GPS alt [m]','texmode','on')
      | port_label('output',10,'Velocity [m/s]')
      | port_label('output',11,'Heading [deg]')
      | port_label('output',12,'Yaw rate [deg/s]')
  STATE_BMW_X5_SUV_1_rc : RateTransition  Tag=mux_rc/StatePort  OutPortSampleTimeOpt=Inherit
  Scope : Scope
  Sensing : Constant
  SimulinkState : Constant  Value=100
  Ssmp : Constant
  Switch : Constant
  a : Constant  Value=0.01
  b : Constant  Value=0.6
  percent_reflecting_sfc : Constant  Value=0.9
  power : Constant  Value=15
  radarDetections : adeye_lib/radarDetections  SystemSampleTime=-1
  z_max : Constant  Value=150
  STATE_BMW_X5_SUV_1_bus : Outport  Tag=outport/StatePort  OutDataTypeStr=Bus: PRESCAN_STATEACTUATORDATA  PortDimensions=1  SampleTime=1/20
  tag scope: other=global, x_value=global
  wires:
  FakeLocalization/1 -> ROS Send Simulink State/5
  Constant33/1 -> Lidar Adapter1/1
  Rviz/1 -> ROS Send Simulink State/1
  Constant2/1 -> Car to Base_link/2
  PointCloudSensor_1_Range_Demux/1(Range) -> Fault Injection Lidar/1
  Lidar Adapter/1 -> [L1]
  Frequency evaluator3/1(Out1) -> [clock]
  Constant/1 -> Lidar Adapter/1
  Constant27/1 -> Relational Operator1/2
  [car_pose] -> Car to Base_link/1
  Frequency evaluator4/1(Out1) -> [state]
  Clock2/1 -> Relational Operator1/1
  Bus Selector1/4 -> Fault Injection Radar/4  "<TargetTypeID[-]>"
  [Roty] -> Car_Pose/5
  Fault Injection Radar/1 -> radarDetections/1
  [Rotx] -> Car_Pose/4
  [x] -> Car_Pose/1
  Car_Pose/1 -> [car_pose]
  [RADAR] -> Bus Selector1/1
  Bus Selector1/2 -> Fault Injection Radar/2  "<Theta[deg]>"
  PointCloudSensor_3_Angles_Demux/2(Phi) -> Fault Injection Lidar2/3
  PointCloudSensor_4_Intensity_Demux/1(Intensity) -> Fault Injection Lidar3/4
  [y] -> Car_Pose/2
  CurrentVelocity/1 -> Frequency evaluator5/1(In1)
  PointCloudSensor_2_Intensity_Demux/1(Intensity) -> Fault Injection Lidar1/4
  Frequency evaluator6/1(Out1) -> [x_value]
  PointCloudSensor_3_Intensity_Demux/1(Intensity) -> Fault Injection Lidar2/4
  Constant34/1 -> Lidar Adapter2/1
  MotionPlanning/1 -> ROS Send Simulink State/8
  MissionPlanning/1 -> ROS Send Simulink State/7
  Frequency evaluator1/1(Out1) -> [points]
  Constant35/1 -> Lidar Adapter3/1
  PointCloudSensor_4_Range_Demux/1(Range) -> Fault Injection Lidar3/1
  PointCloudSensor_3_Angles_Demux/1(Theta) -> Fault Injection Lidar2/2
  [other] -> radarDetections/Enable
  PointCloudSensor_4_Angles_Demux/2(Phi) -> Fault Injection Lidar3/3
  [velocity] -> ROS Send Odometry/2
  PointCloudSensor_2_Range_Demux/1(Range) -> Fault Injection Lidar1/1
  Constant8/1 -> Fault Injection Camera/4
  [yaw_rate] -> ROS Send Odometry/3
  PointCloudSensor_2_Angles_Demux/1(Theta) -> Fault Injection Lidar1/2
  ImageRaw/1 -> Frequency evaluator2/1(In1)
  ? -> Distance_evaluator/1(In1)
  SELF_Demux/11(heading [deg]) -> ?
  Constant9/1 -> Fault Injection Radar/5
  SELF_Demux/8(GPS long [deg]) -> ?
  PointCloudSensor_2_Angles_Demux/2(Phi) -> Fault Injection Lidar1/3
  Constant6/1 -> Car to Base_link/3
  SELF_Demux/9(GPS alt [m]) -> ?
  GnssPoseSimulink/1 -> Frequency evaluator/1(In1)
  [R] -> Fault Injection Lidar1/5
  Bus Selector1/3 -> Fault Injection Radar/3  "<Phi[deg]>"
  PointCloudSensor_1_Angles_Demux/2(Phi) -> Fault Injection Lidar/3
  [B3] -> ROS Send Camera 2/3
  Fault Injection Radar/3 -> radarDetections/3
  Localization/1 -> ROS Send Simulink State/4
  Lidar Adapter3/1 -> [L4]
  [z_max] -> Fault Injection Lidar1/10
  PointsRawFloat32/1 -> Frequency evaluator1/1(In1)
  SELF_Demux/7(GPS lat [deg]) -> ?
  PointCloudSensor_4_Angles_Demux/1(Theta) -> Fault Injection Lidar3/2
  [power] -> Fault Injection Lidar/8
  [clock] -> ROS Send Clock/Enable
  Constant15/1 -> Fault Injection Lidar3/11
  GoalDistance/1 -> Distance_evaluator/3(In3)
  [state] -> ROS Send Simulink State/Enable
  Frequency evaluator5/1(Out1) -> [vel]
  PoseOtherCar/1 -> Frequency evaluator7/1(In1)
  [vel] -> ROS Send Velocity/Enable
  [power] -> Fault Injection Lidar1/8
  PointCloudSensor_3_Range_Demux/1(Range) -> Fault Injection Lidar2/1
  GoalOrientW/1 -> ROS Send Goal/4
  Sensing/1 -> ROS Send Simulink State/3
  [base_link_pose] -> ROS Send Odometry/1
  [B1] -> ROS Send Camera/3
  [b] -> Fault Injection Lidar2/7
  GoalPoseX/1 -> ROS Send Goal/1
  Lidar Adapter2/1 -> [L3]
  Switch/1 -> ROS Send Simulink State/9
  GoalPoseY/1 -> ROS Send Goal/2
  [power] -> Fault Injection Lidar3/8
  Ssmp/1 -> ROS Send Simulink State/10
  Constant10/1 -> Fault Injection Lidar/11
  Fault Injection Lidar3/4 -> Lidar Adapter3/5
  SELF_Demux/10(velocity [m/s]) -> Scope/1, Dynamics_Empty/1(In1), [velocity]
  [a] -> Fault Injection Lidar3/6
  [p_refl_sfc] -> Fault Injection Lidar/9
  [R] -> Fault Injection Lidar2/5
  [base_link_pose] -> Fault Injection GNSS/1
  Fault Injection Lidar1/4 -> Lidar Adapter1/5
  power/1 -> [power]
  Fault Injection Lidar2/2 -> Lidar Adapter2/3
  ClockFrequency/1 -> Frequency evaluator3/1(In1)
  [a] -> Fault Injection Lidar1/6
  [p_refl_sfc] -> Fault Injection Lidar1/9
  PointCloudSensor_1_Intensity_Demux/1(Intensity) -> Fault Injection Lidar/4
  Frequency evaluator2/1(Out1) -> [image]
  [yaw_rate] -> ROS Send Velocity/2
  [Rotx] -> ROS Send IMU/1
  Fault Injection Lidar3/2 -> Lidar Adapter3/3
  [R] -> Fault Injection Lidar3/5
  Constant12/1 -> ROS Send Switch Command/Enable
  Lidar Adapter1/1 -> [L2]
  Fault Injection Radar/2 -> radarDetections/2
  [z_max] -> Fault Injection Lidar2/10
  Constant11/1 -> ROS Send Switch Command/1
  Fault Injection Lidar3/1 -> Lidar Adapter3/2
  Constant14/1 -> Fault Injection Lidar2/11
  [velocity] -> ROS Send Velocity/1
  Fault Injection Lidar2/1 -> Lidar Adapter2/2
  [z] -> Car_Pose/3
  [p_refl_sfc] -> Fault Injection Lidar3/9
  [z_max] -> Fault Injection Lidar3/10
  percent_reflecting_sfc/1 -> [p_refl_sfc]
  Fault Injection Lidar3/3 -> Lidar Adapter3/4
  SELF_Demux/3(z [m]) -> [z]
  Detection/1 -> ROS Send Simulink State/6
  Fault Injection Lidar2/4 -> Lidar Adapter2/5
  SELF_Demux/1(x [m]) -> [x]
  Fault Injection Lidar/1 -> Lidar Adapter/2
  [power] -> Fault Injection Lidar2/8
  [image] -> ROS Send Camera/Enable
  Fault Injection Lidar1/1 -> Lidar Adapter1/2
  [a] -> Fault Injection Lidar/6
  Fault Injection Lidar/3 -> Lidar Adapter/4
  GoalOrientZ/1 -> ROS Send Goal/7
  CurrentPose/1 -> Frequency evaluator6/1(In1)
  Fault Injection Lidar/4 -> Lidar Adapter/5
  R/1 -> [R]
  [z_max] -> Fault Injection Lidar/10
  Frequency evaluator/1(Out1) -> [gnss]
  GoalOrientX/1 -> ROS Send Goal/5
  [R] -> Fault Injection Lidar/5
  [p_refl_sfc] -> Fault Injection Lidar2/9
  z_max/1 -> [z_max]
  [b] -> Fault Injection Lidar3/7
  SELF_Demux/12(yaw rate [deg/s]) -> [yaw_rate]
  GoalOrientY/1 -> ROS Send Goal/6
  a/1 -> [a]
  [velocity] -> ROS Send IMU/5
  [b] -> Fault Injection Lidar/7
  Fault Injection Lidar/2 -> Lidar Adapter/3
  Map/1 -> ROS Send Simulink State/2
  [R1] -> ROS Send Camera/1
  Constant13/1 -> Fault Injection Lidar1/11
  Car to Base_link/1 -> [base_link_pose]
  Constant1/1 -> Fault Injection GNSS/2
  [b] -> Fault Injection Lidar1/7
  SELF_Demux/2(y [m]) -> [y]
  [points] -> ROS Send Lidar/Enable
  Relational Operator1/1 -> ROS Send Goal/Enable
  [R3] -> ROS Send Camera 2/1
  Fault Injection GNSS/1 -> ROS Send GNSS/1
  Fault Injection Lidar1/3 -> Lidar Adapter1/4
  [Rotz] -> ROS Send IMU/3
  SELF_Demux/5(roty [deg]) -> [Roty]
  [L3] -> ROS Send Lidar/3
  [other] -> ROS Send IMU/Enable
  [yaw_rate] -> ROS Send IMU/4
  [G2] -> ROS Send Camera TL/2
  [G3] -> ROS Send Camera 2/2
  [a] -> Fault Injection Lidar2/6
  GoalPoseZ/1 -> ROS Send Goal/3
  From6/1 -> Distance_evaluator/2(In2)
  Clock/1 -> ROS Send Clock/1
  SELF_Demux/4(rotx [deg]) -> [Rotx]
  Constant7/1 -> Car to Base_link/4
  Frequency evaluator7/1(Out1) -> [other]
  b/1 -> [b]
  [R2] -> ROS Send Camera TL/1
  [Rotz] -> Car_Pose/6
  [G1] -> ROS Send Camera/2
  [L4] -> ROS Send Lidar/4
  Bus Selector1/1 -> Fault Injection Radar/1  "<Range[m]>"
  PointCloudSensor_1_Angles_Demux/1(Theta) -> Fault Injection Lidar/2
  Fault Injection Lidar2/3 -> Lidar Adapter2/4
  [image] -> ROS Send Camera 2/Enable
  Radar_1_Demux/1(Radar Data) -> [RADAR]
  [gnss] -> ROS Send GNSS/Enable
  Fault Injection Lidar1/2 -> Lidar Adapter1/3
  [B2] -> ROS Send Camera TL/3
  Fault Injection Radar/4 -> radarDetections/4
  Constant20/1 -> ROS Send Odometry/Enable
  [Roty] -> ROS Send IMU/2
  SELF_Demux/6(rotz [deg]) -> [Rotz]
  [image] -> ROS Send Camera TL/Enable
  SimulinkState/1 -> Frequency evaluator4/1(In1)
  [L2] -> ROS Send Lidar/2
  [L1] -> ROS Send Lidar/1
  Camera_1_CM_Demux/3(B) -> [B1], Camera_1_CM_Display/3
  Camera_2_CM_Demux/2(G) -> [G3], Camera_2_CM_Display/2
  Camera_2_CM_Demux/1(R) -> [R3], Camera_2_CM_Display/1
  Camera_1_CM_Demux/2(G) -> [G1], Camera_1_CM_Display/2
  Camera_tl_CM_Demux/1(R) -> [R2], Camera_tl_CM_Display/1
  Camera_2_CM_Demux/3(B) -> [B3], Camera_2_CM_Display/3
  Camera_1_CM_Demux/1(R) -> [R1], Camera_1_CM_Display/1
  Camera_tl_CM_Demux/3(B) -> [B2], Camera_tl_CM_Display/3
  Camera_tl_CM_Demux/2(G) -> [G2], Camera_tl_CM_Display/2
  STATE_BMW_X5_SUV_1_rc/1 -> STATE_BMW_X5_SUV_1_bus/1
  SELF_BMW_X5_SUV_1/1 -> SELF_Demux/1(SELF)
  Radar_1/1 -> Radar_1_Demux/1(Radar)
  PointCloudSensor_1/1 -> PointCloudSensor_1_Range_Demux/1(In1), PointCloudSensor_1_Angles_Demux/1(In2), PointCloudSensor_1_Intensity_Demux/1(In1)
  PointCloudSensor_2/1 -> PointCloudSensor_2_Range_Demux/1(In1), PointCloudSensor_2_Angles_Demux/1(In2), PointCloudSensor_2_Intensity_Demux/1(In1)
  PointCloudSensor_3/1 -> PointCloudSensor_3_Range_Demux/1(In1), PointCloudSensor_3_Angles_Demux/1(In2), PointCloudSensor_3_Intensity_Demux/1(In1)
  PointCloudSensor_4/1 -> PointCloudSensor_4_Range_Demux/1(In1), PointCloudSensor_4_Angles_Demux/1(In2), PointCloudSensor_4_Intensity_Demux/1(In1)
  Camera_1/1 -> Camera_1_CM_Demux/1(In1)
  Camera_tl/1 -> Camera_tl_CM_Demux/1(In1)
  HumViewCamera/1 -> HumViewCamera_CM_Demux/1(In1)
  HumViewCamera_CM_Demux/1(R) -> HumViewCamera_CM_Display/1
  HumViewCamera_CM_Demux/2(G) -> HumViewCamera_CM_Display/2
  HumViewCamera_CM_Demux/3(B) -> HumViewCamera_CM_Display/3
  Camera_2/1 -> Camera_2_CM_Demux/1(In1)
  Dynamics_Empty/1(State) -> STATE_BMW_X5_SUV_1_rc/1

== system Experiment_cs/Camera_1 ==
  Sensor : S-Function  FunctionName=sfun_Camera  Parameters=sensorID, dataWidth, dataHeight, channelsPerImage, numberOfImages, timestep  SFunctionDeploymentMode=off  EnableBusSupport=off  mask(PreScan Source Block: Camera Sensor){sensorID=261, dataWidth=720, dataHeight=2880, channelsPerImage=3, numberOfImages=1, timestep=1/20}
      mask prompts: sensorID "Sensor ID"; dataWidth "Data width"; dataHeight "Data Height"; channelsPerImage "Channels per image"; numberOfImages "Number of images"; timestep "MATLAB timestep:"
      mask help: The Camera Sensor provides a color or monochrome image.
      mask Help: eval('openHelp(457)')
      mask Display: image(imread('CameraSensor.png'))
  Camera_1 : Outport  Tag=outport/Camera/CameraSensor  OutDataTypeStr=uint8  SampleTime=1/20
  wires:
  Sensor/1 -> Camera_1/1

== system Experiment_cs/Camera_2 ==
  Sensor : S-Function  FunctionName=sfun_Camera  Parameters=sensorID, dataWidth, dataHeight, channelsPerImage, numberOfImages, timestep  SFunctionDeploymentMode=off  EnableBusSupport=off  mask(PreScan Source Block: Camera Sensor){sensorID=265, dataWidth=720, dataHeight=2880, channelsPerImage=3, numberOfImages=1, timestep=1/20}
      mask prompts: sensorID "Sensor ID"; dataWidth "Data width"; dataHeight "Data Height"; channelsPerImage "Channels per image"; numberOfImages "Number of images"; timestep "MATLAB timestep:"
      mask help: The Camera Sensor provides a color or monochrome image.
      mask Help: eval('openHelp(457)')
      mask Display: image(imread('CameraSensor.png'))
  Camera_2 : Outport  Tag=outport/Camera/CameraSensor  OutDataTypeStr=uint8  SampleTime=1/20
  wires:
  Sensor/1 -> Camera_2/1

== system Experiment_cs/Camera_tl ==
  Sensor : S-Function  FunctionName=sfun_Camera  Parameters=sensorID, dataWidth, dataHeight, channelsPerImage, numberOfImages, timestep  SFunctionDeploymentMode=off  EnableBusSupport=off  mask(PreScan Source Block: Camera Sensor){sensorID=262, dataWidth=720, dataHeight=2880, channelsPerImage=3, numberOfImages=1, timestep=1/20}
      mask prompts: sensorID "Sensor ID"; dataWidth "Data width"; dataHeight "Data Height"; channelsPerImage "Channels per image"; numberOfImages "Number of images"; timestep "MATLAB timestep:"
      mask help: The Camera Sensor provides a color or monochrome image.
      mask Help: eval('openHelp(457)')
      mask Display: image(imread('CameraSensor.png'))
  Camera_tl : Outport  Tag=outport/Camera/CameraSensor  OutDataTypeStr=uint8  SampleTime=1/20
  wires:
  Sensor/1 -> Camera_tl/1

== system Experiment_cs/Controller ==
  Terminator : Terminator
  sfun_Controller : S-Function  FunctionName=sfun_Controller  Parameters=SParameter1, SParameter2, SParameter3, SParameter4, SParameter5, SParameter6, SParameter7, SParameter8, SParameter9, SParameter10, SampleTime  SFunctionDeploymentMode=off  EnableBusSupport=off  mask(Legacy Function){SFunctionSpec=void prescan_outputFcn(void** work1, PRESCAN_CONTROLLERDATA y1[1]), SParameter1=uint8([ExperimentFile 0]), SParameter2=uint8([ModelDepo 0]), SParameter3=uint8([ControllerOptions 0]), SParameter4=RTmode, SParameter5=PreScanExecutionMode, SParameter6=ControlMode, SParameter7=ControllerCount, SParameter8=ControllerIndex, SParameter9=uint8([SimulationMode 0]), SParameter10=uint8([TargetName 0]), SampleTime=TimeStep, ShowSpec=on}
      mask prompts: SParameter1 "P1:"; SParameter2 "P2:"; SParameter3 "P3:"; SParameter4 "P4:"; SParameter5 "P5:"; SParameter6 "P6:"; SParameter7 "P7:"; SParameter8 "P8:"; SParameter9 "P9:"; SParameter10 "P10:"; SampleTime "Sample time (-1 for inherited):"; ShowSpec "Display function specification"
      mask help:
      | This block allows you to call the legacy functions specified by the following Legacy Code Tool definition:
      | def.SFunctionName = 'sfun_Controller';
      | def.OutputFcnSpec = 'void prescan_outputFcn(void** work1, PRESCAN_CONTROLLERDATA y1[1])';
      | def.StartFcnSpec = 'void prescan_startFcn(void ** work1, uint8 p1[], uint8 p2[], uint8 p3[], double p4, double p5, double p6, double p7, double p8, uint8 p9[], uint8 p10[])';
      | def.TerminateFcnSpec = 'void prescan_terminateFcn(void** work1)';
      | def.HeaderFiles = {'prescan_controller_data.h', 'prescan_SFunLibrary.h', 'prescan_CreateLogHandler.h', 'prescan_CreateErrorHandler.h', 'prescan_modify.h', 'ModuleDLL.h'};
      | def.SourceFiles = {'prescan_MexLogHandler.c', 'prescan_SimStructErrorHandler.c', 'prescan_LogHandler.c', 'prescan_ErrorHandler.c', 'prescan_Modify.c'};
      | def.HostLibFiles = {'sensorinterfaced.lib'};
      | def.TargetLibFiles = {'sensorinterfaced.so'};
      | def.IncPaths = {'.', 'C:\projects\prescan\rt_vislibrary\vis\..\pimp\include\sensors\InterfaceRTW'};
      | def.SrcPaths = {'C:\projects\prescan\rt_vislibrary\vis\..\pimp\include\sensors\InterfaceRTW', 'C:\projects\prescan\rt_vislibrary\vis\..\pimp\include\sensors\InterfaceRTW\ccurrt'};
      | def.LibPaths = {'C:\\projects\\prescan\\vislibrary_build\lib'};
      | def.SampleTime = 'parameterized';
      mask Help: <p>This block was generated automatically by the Legacy Code Tool. For detailed help on this tool, call<a href="matlab:legacy_code('help')"> legacy_code('help')</a>.</p>
      mask Callback ShowSpec:
      | if strcmp(get_param(gcbh, 'ShowSpec'), 'on')
      |   set_param(gcbh, 'MaskDisplay', sprintf('fprintf(''%s'');', get_param(gcbh, 'SFunctionSpec')));
      | else
      |   set_param(gcbh, 'MaskDisplay', sprintf('fprintf(''%s'');', get_param(gcbh, 'FunctionName')));
      | end
      mask Display: fprintf('void prescan_outputFcn(void** work1, PRESCAN_CONTROLLERDATA y1[1])');
  wires:
  sfun_Controller/1 -> Terminator/1
